simulink model "GaNCore"  (R2016a)
settings: Solver=VariableStepAuto  StartTime=0.0  StopTime=10.0  RelTol=1e-3
libraries: fl_lib x14, nesl_utility x6
settings Model: Creator=enes_  LastModifiedBy=enes_

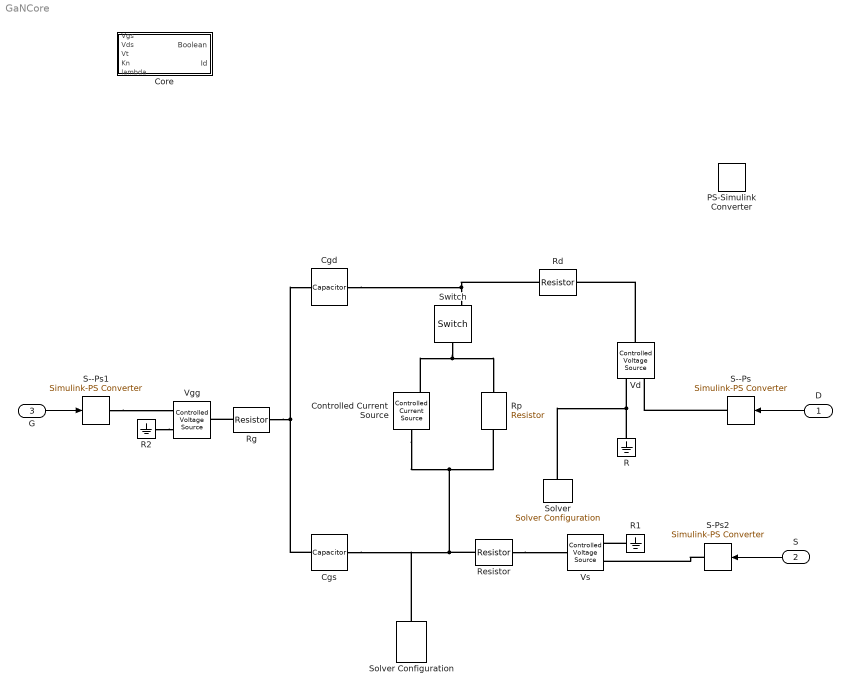
== system GaNCore ==
  D : Inport
  S : Inport  Port=2
  G : Inport  Port=3
  Cgd : fl_lib/Electrical/Electrical Elements/Capacitor  c=1e-6 F  r=1e-6 Ohm  g=0 1/Ohm  i_specify=off  i_priority=None  i=0 A  v_specify=off  v_priority=None  v=0 V  vc_specify=off  vc_priority=High  vc=0 V
  Cgs : fl_lib/Electrical/Electrical Elements/Capacitor  c=1e-6 F  r=1e-6 Ohm  g=0 1/Ohm  i_specify=off  i_priority=None  i=0 A  v_specify=off  v_priority=None  v=0 V  vc_specify=off  vc_priority=High  vc=0 V
  Controlled Current Source : fl_lib/Electrical/Electrical Sources/Controlled Current Source
  Core : Subsystem
  PS-Simulink Converter : nesl_utility/PS-Simulink Converter  PhysicalDomain=network_engine_domain  SubClassName=ps_output  LeftPortType=input  RightPortType=output  PseudoPeriodic=off  Frequencies=[]  Unit=1  AffineConversion=off
  R : fl_lib/Electrical/Electrical Elements/Electrical Reference
  R1 : fl_lib/Electrical/Electrical Elements/Electrical Reference
  R2 : fl_lib/Electrical/Electrical Elements/Electrical Reference
  Rd : fl_lib/Electrical/Electrical Elements/Resistor  R=1 Ohm  i_specify=off  i_priority=None  i=0 A  v_specify=off  v_priority=None  v=0 V
  Resistor : fl_lib/Electrical/Electrical Elements/Resistor  R=1 Ohm  i_specify=off  i_priority=None  i=0 A  v_specify=off  v_priority=None  v=0 V
  Rg : fl_lib/Electrical/Electrical Elements/Resistor  R=1 Ohm  i_specify=off  i_priority=None  i=0 A  v_specify=off  v_priority=None  v=0 V
  Rp : fl_lib/Electrical/Electrical Elements/Resistor  R=1 Ohm  i_specify=off  i_priority=None  i=0 A  v_specify=off  v_priority=None  v=0 V
  S--Ps : nesl_utility/Simulink-PS Converter  PhysicalDomain=network_engine_domain  SubClassName=ps_input  LeftPortType=input  RightPortType=output  PseudoPeriodic=off  Frequencies=[]  NoiseDistribution=none  NoiseParameters=[]  Unit=1  AffineConversion=off  InputFiltering=off  SimscapeFilterOrder=1  InputFilterTimeConstant=0.001  UdotUserProvided=1
  S--Ps1 : nesl_utility/Simulink-PS Converter  PhysicalDomain=network_engine_domain  SubClassName=ps_input  LeftPortType=input  RightPortType=output  PseudoPeriodic=off  Frequencies=[]  NoiseDistribution=none  NoiseParameters=[]  Unit=1  AffineConversion=off  InputFiltering=off  SimscapeFilterOrder=1  InputFilterTimeConstant=0.001  UdotUserProvided=1
  S-Ps2 : nesl_utility/Simulink-PS Converter  PhysicalDomain=network_engine_domain  SubClassName=ps_input  LeftPortType=input  RightPortType=output  PseudoPeriodic=off  Frequencies=[]  NoiseDistribution=none  NoiseParameters=[]  Unit=1  AffineConversion=off  InputFiltering=off  SimscapeFilterOrder=1  InputFilterTimeConstant=0.001  UdotUserProvided=1
  Solver : nesl_utility/Solver Configuration  PhysicalDomain=network_engine_domain  SubClassName=solver  LeftPortType=input  RightPortType=generic  Accelerate=off  Tones=[]  Harmonics=[]  SimulateNoise=off  Profile=off  UseLocalSampling=off  EnableSwitchedLinearOptims=on  FrequencyDomain=off  UseCCode=off  RelTol=0.001  AbsTol=1e-06  MinStep=1e-09  ToWorkspace=off  RevertToSquareIcSolve=off  NumHomotopyIterations=100  PhasorMode=off  PhasorModeNumHarmonics=1  OverrideAbsTol=off  DoDC=off  ResidualTolerance=1e-09  UseLocalSolver=off  LocalSolverChoice=NE_BACKWARD_EULER_ADVANCER  LocalSolverSampleTime=0.001  DoFixedCost=off  MaxNonlinIter=3  MaxModeIter=2  LinearAlgebra=Sparse  DelaysMemoryBudget=1024  AutomaticFiltering=on  FilteringTimeConstant=0.001
  Solver Configuration : nesl_utility/Solver Configuration  PhysicalDomain=network_engine_domain  SubClassName=solver  LeftPortType=input  RightPortType=generic  Accelerate=off  Tones=[]  Harmonics=[]  SimulateNoise=off  Profile=off  UseLocalSampling=off  EnableSwitchedLinearOptims=on  FrequencyDomain=off  UseCCode=off  RelTol=0.001  AbsTol=1e-06  MinStep=1e-09  ToWorkspace=off  RevertToSquareIcSolve=off  NumHomotopyIterations=100  PhasorMode=off  PhasorModeNumHarmonics=1  OverrideAbsTol=off  DoDC=off  ResidualTolerance=1e-09  UseLocalSolver=off  LocalSolverChoice=NE_BACKWARD_EULER_ADVANCER  LocalSolverSampleTime=0.001  DoFixedCost=off  MaxNonlinIter=3  MaxModeIter=2  LinearAlgebra=Sparse  DelaysMemoryBudget=1024  AutomaticFiltering=on  FilteringTimeConstant=0.001
  Switch : fl_lib/Electrical/Electrical Elements/Switch  R_closed=0.01 Ohm  G_open=1e-8 1/Ohm  Threshold=0  i_specify=off  i_priority=None  i=0 A  v_specify=off  v_priority=None  v=0 V
  Vd : fl_lib/Electrical/Electrical Sources/Controlled Voltage Source
  Vgg : fl_lib/Electrical/Electrical Sources/Controlled Voltage Source
  Vs : fl_lib/Electrical/Electrical Sources/Controlled Voltage Source
  wires:
  D/1 -> S--Ps/1
  S/1 -> S-Ps2/1
  G/1 -> S--Ps1/1
  connections:
  Vd/LConn1 -- Rd/LConn1
  R/LConn1 -- Vd/RConn2 -- Solver/RConn1
  S--Ps/RConn1 -- Vd/RConn1
  Rd/RConn1 -- Cgd/LConn1 -- Switch/RConn2
  Switch/LConn1 -- Rp/LConn1 -- Controlled Current Source/RConn2
  Controlled Current Source/LConn1 -- Cgs/RConn1 -- Solver Configuration/RConn1 -- Resistor/LConn1 -- Rp/RConn1
  Resistor/RConn1 -- Vs/LConn1
  R1/LConn1 -- Vs/RConn2
  S-Ps2/RConn1 -- Vs/RConn1
  S--Ps1/RConn1 -- Vgg/RConn1
  R2/LConn1 -- Vgg/RConn2
  Rg/LConn1 -- Vgg/LConn1
  Rg/RConn1 -- Cgd/RConn1 -- Cgs/LConn1

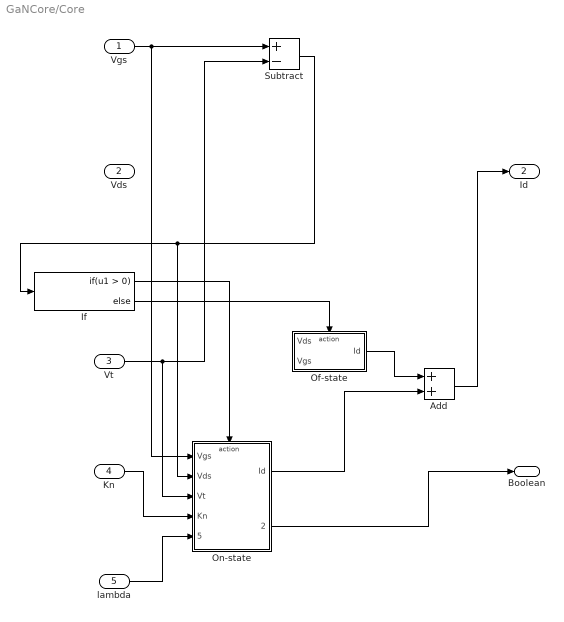
== system GaNCore/Core ==
  Vgs : Inport
  Vds : Inport  Port=2
  Vt : Inport  Port=3
  Kn : Inport  Port=4
  lambda : Inport  Port=5
  Add : Sum
  If : If
  Of-state : Subsystem  TreatAsAtomicUnit=on
  On-state : Subsystem  TreatAsAtomicUnit=on
  Subtract : Sum  Inputs=+-
  Boolean : Outport
  Id : Outport  Port=2
  wires:
  If/1 -> On-state/Action
  If/2 -> Of-state/Action
  Vgs/1 -> Subtract/1, On-state/1(Vgs)
  Vt/1 -> On-state/3(Vt), Subtract/2
  Subtract/1 -> On-state/2(Vds), If/1
  Of-state/1(Id) -> Add/1
  On-state/1(Id) -> Add/2
  Add/1 -> Id/1
  On-state/2(Boolean) -> Boolean/1
  Kn/1 -> On-state/4(Kn)
  lambda/1 -> On-state/5(lambda)

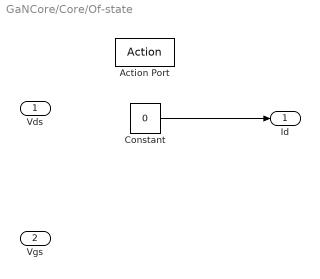
== system GaNCore/Core/Of-state ==
  Vds : Inport
  Vgs : Inport  Port=2
  Action Port : ActionPort  ActionType=else
  Constant : Constant  Value=0
  Id : Outport
  wires:
  Constant/1 -> Id/1

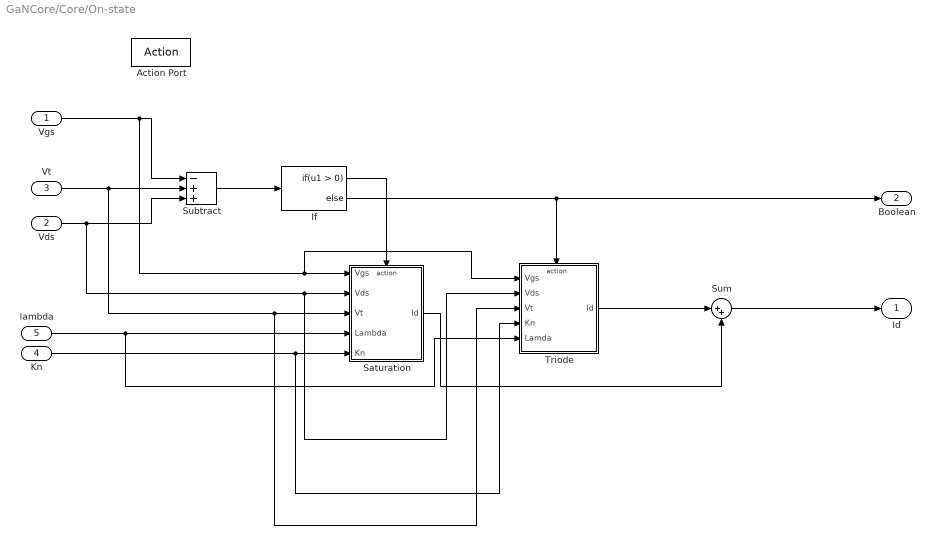
== system GaNCore/Core/On-state ==
  Vgs : Inport
  Vds : Inport  Port=2
  Vt : Inport  Port=3
  Kn : Inport  Port=4
  lambda : Inport  Port=5
  Action Port : ActionPort  ActionType=then
  If : If
  Saturation : Subsystem  TreatAsAtomicUnit=on
  Subtract : Sum  Inputs=-++
  Sum : Sum  Inputs=|++
  Triode : Subsystem  TreatAsAtomicUnit=on
  Id : Outport
  Boolean : Outport  Port=2
  wires:
  Vds/1 -> Triode/2(Vds), Saturation/2(Vds), Subtract/3
  Subtract/1 -> If/1
  If/1 -> Saturation/Action
  If/2 -> Boolean/1, Triode/Action
  Vgs/1 -> Triode/1(Vgs), Saturation/1(Vgs), Subtract/1
  Vt/1 -> Triode/3(Vt), Saturation/3("Vt "), Subtract/2
  Kn/1 -> Triode/4(Kn), Saturation/5(Kn)
  lambda/1 -> Triode/5(Lamda), Saturation/4(Lambda)
  Triode/1(Id) -> Sum/1
  Saturation/1(Id) -> Sum/2
  Sum/1 -> Id/1

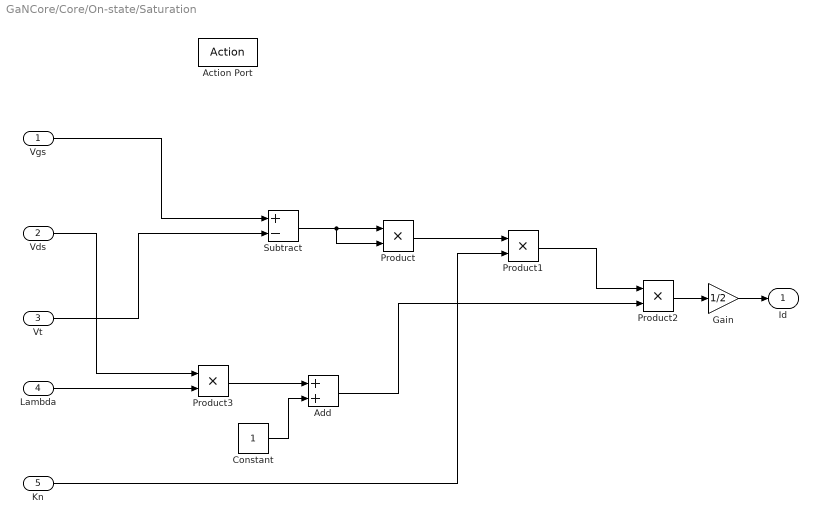
== system GaNCore/Core/On-state/Saturation ==
  Vgs : Inport
  Vds : Inport  Port=2
  "Vt " : Inport  Port=3
  Lambda : Inport  Port=4
  Kn : Inport  Port=5
  Action Port : ActionPort  ActionType=then
  Add : Sum
  Constant : Constant
  Gain : Gain  Gain=1/2
  Product{,1..3} (4 alike) : Product
  Subtract : Sum  Inputs=+-
  Id : Outport
  wires:
  Vgs/1 -> Subtract/1
  "Vt "/1 -> Subtract/2
  Subtract/1 -> Product/2, Product/1
  Kn/1 -> Product1/2
  Vds/1 -> Product3/1
  Lambda/1 -> Product3/2
  Product3/1 -> Add/1
  Constant/1 -> Add/2
  Add/1 -> Product2/2
  Product1/1 -> Product2/1
  Product2/1 -> Gain/1
  Product/1 -> Product1/1
  Gain/1 -> Id/1

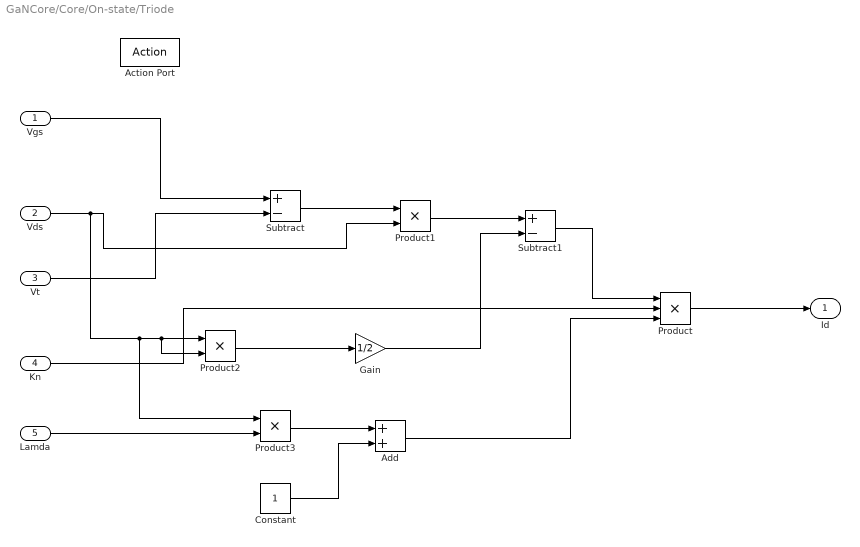
== system GaNCore/Core/On-state/Triode ==
  Vgs : Inport
  Vds : Inport  Port=2
  Vt : Inport  Port=3
  Kn : Inport  Port=4
  Lamda : Inport  Port=5
  Action Port : ActionPort  ActionType=else
  Add : Sum
  Constant : Constant
  Gain : Gain  Gain=1/2
  Product : Product  Inputs=3
  Product1 : Product
  Product2 : Product
  Product3 : Product
  Subtract : Sum  Inputs=+-
  Subtract1 : Sum  Inputs=+-
  Id : Outport
  wires:
  Vgs/1 -> Subtract/1
  Vt/1 -> Subtract/2
  Subtract/1 -> Product1/1
  Product1/1 -> Subtract1/1
  Product2/1 -> Gain/1
  Gain/1 -> Subtract1/2
  Vds/1 -> Product1/2, Product3/1, Product2/2, Product2/1
  Lamda/1 -> Product3/2
  Product3/1 -> Add/1
  Constant/1 -> Add/2
  Subtract1/1 -> Product/1
  Kn/1 -> Product/2
  Add/1 -> Product/3
  Product/1 -> Id/1
